simulink model "visual_line_follower_sac_residual"  (R2026a)
settings: Solver=FixedStepDiscrete  StopTime=40  FixedStep=MJ_StepTime  EnableMultiTasking=on
InitFcn:
  | run(fullfile(fileparts(get_param(bdroot,"FileName")),"runtime","init","configure_turtlebot3_visual_line_follower_paths.m"));
model workspace (MAT data in the model file):
  BaseLinearSpeed = 5
  BaseSpeedScale = 0.03
  Kd_Line = 0.35
  Ki_Line = 0
  Kp_Line = 5
  LocalPath_CurvatureGain = 0.04
  LocalPath_HeadingGain = 0.35
  LocalPath_LateralGain = 0.6
  LocalPath_LookaheadDistance = 0.2
  LocalPath_NumPoints = 30
  LocalPath_ROIFraction = 0.3
  MJ_StepTime = 0.002
  MJ_TargetLateralPosition = 0
  MaxAngularSpeed = 1.5
  MaxWheelSpeed = 7.9
  N_Line = 20
  OriginBot_ErrorScale = 500
  OriginBot_MaxSaturation = 0.3
  OriginBot_MinBrightness = 70
  OriginBot_MinPixels = 30
  OriginBot_ROIHeight = 45
  OriginBot_ROIStartFraction = 0.72
  SAC_Done_Steps = 100
  SAC_MaxDeltaOmega = 1
  SAC_MaxDeltaV = 1
  SAC_P_Lost = 10
  SAC_Q = 1
  SAC_Q_Heading = 0.5
  SAC_Q_Lateral = 0.5
  SAC_R = 0.1
  Safety_BrakeTime = 0.3
  Safety_CBFAlpha = 2
  Safety_CBFSingularTol = 0.001
  Safety_DirDeadband = 0.02
  Safety_EnableFilter = 1
  Safety_EnableSearch = 0
  Safety_HoldTime = 0.4
  Safety_LateralMax = 0.8
  Safety_MaxAccelOmega = 10
  Safety_MaxAccelV = 40
  Safety_MemLookahead = 0.25
  Safety_MemMaxAge = 8
  Safety_MemMinPoints = 3
  Safety_RecoverAlignCone = 0.785398163397
  Safety_RecoverGain = 1.5
  Safety_RecoverSpeedFrac = 0.25
  Safety_RecoverTimeout = 8
  Safety_ScanAmplitudes = [0.436332312999 0.872664625997 1.3962634016]
  Safety_ScanRate = 0.9
  Safety_ScanTimeout = 15
  Safety_ScanTolerance = 0.05
  Safety_SpeedBackoff = 0.3
  SteeringSign = -1
  TB3_WheelRadius = 0.033
  TB3_WheelSeparation = 0.16
  Ts_Control = 0.05
  Ts_Stop = 10
  Ts_Vision = 0.05
  TurtleBot3MuJoCoMap = "simple"
  TurtleBot3MuJoCoScene = ""
undefined symbols (not defined in the file or in its folder): lf_line_search, LF_Safety, lf_safety_filter, originbot_line_follower_debug_frame, originbot_sliding_window_path_generator
libraries: mjLib x1, slpidlib x1, rllib x1
settings Model: ExtModeTrigDuration=10000  Creator=HP  LastModifiedBy=kevin
settings SolverCC: PositivePriorityOrder=on
settings ConfigComp: CovMetricSettings=dswe

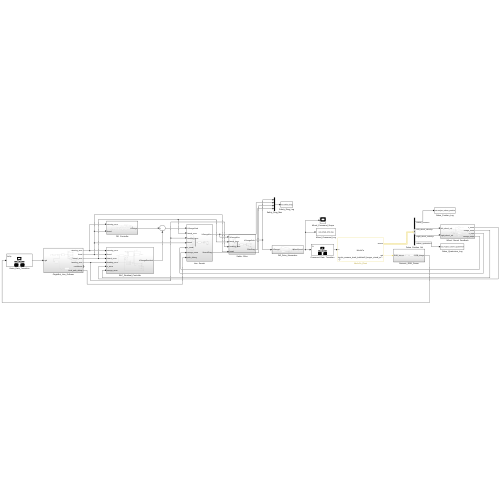
[thumbnail: Simulink's stored preview of the top-level diagram]
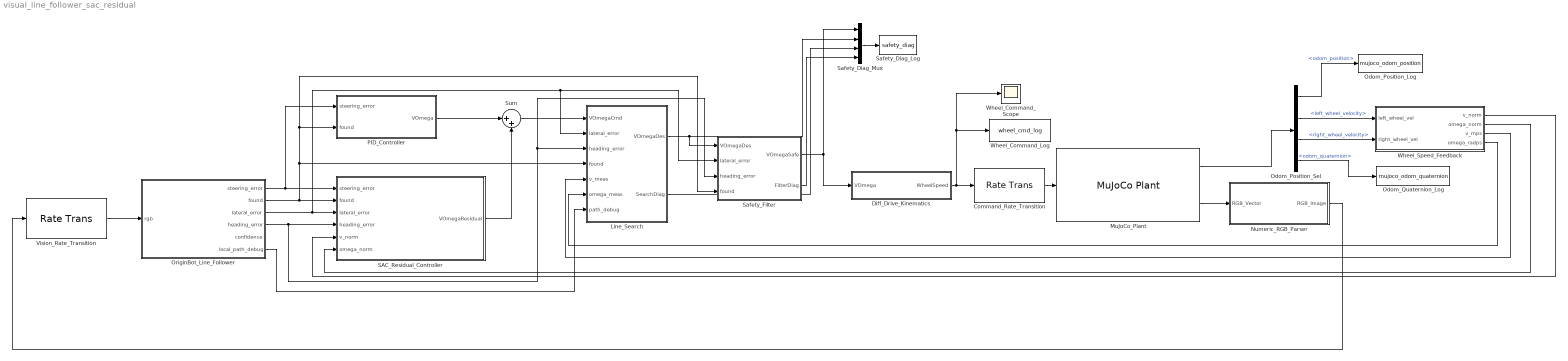
== system visual_line_follower_sac_residual ==
  Command_Rate_Transition : RateTransition  OutPortSampleTime=MJ_StepTime
  Diff_Drive_Kinematics : Subsystem  Description=Shared linear+angular velocity -> left/right wheel-speed converter. Input VOmega=[v;omega] is the summed PID+SAC velocity command (blk_124.y1); output WheelSpeed=[left;right] feeds SAC_PID_Sat (blk_125). Extracted 2026-07-21 from duplicated logic that used to live separately inside PID_Controller and SAC_Residual_Controller -- both now output [v;omega] instead of wheel speeds directly, and this is the ONE place the differential-drive kinematics conversion happens.
  Line_Search : Subsystem
  MuJoCo_Plant : mjLib/MuJoCo Plant  controlBus=[]  sensorBus=mj_bus_sensor_7979902499018342666  controlLength=[]  sensorLength=[]  rgbLength=[]  depthLength=[]  sampleTime=0.002  xmlFileRel=/media/kevin/ding/final_project/Sheffield/for_getting_started/src/simple_camera_pid/matlab/../model/mujoco/turtlebot3/simple_camera_track_turtlebot3_burger_visual_scene.xml  xmlFile=/media/kevin/ding/final_project/Sheffield/for_getting_started/src/simple_camera_pid/matlab/../model/mujoco/turtlebot3/simple_camera_track_turtlebot3_burger_visual_scene.xml  renderingType=Local  vsync=on  visualFPS=60  zoomLevel=1  znear=0.062275  zfar=311.3772  cameraSampleTime=Ts_Vision  rgbOutOption=on  depthOutOption=off  controlInterfaceType=Vector
      settings: SourceProductName=MuJoCo Simulator
  Numeric_RGB_Parser : Subsystem
  Odom_Position_Log : ToWorkspace  VariableName=mujoco_odom_position  SaveFormat=Timeseries  SampleTime=-1
  Odom_Position_Sel : BusSelector  OutputSignals=odom_position,left_wheel_velocity,right_wheel_velocity,odom_quaternion
  Odom_Quaternion_Log : ToWorkspace  VariableName=mujoco_odom_quaternion  SaveFormat=Timeseries  SampleTime=-1
  OriginBot_Line_Follower : Subsystem
  PID_Controller : Subsystem
  SAC_Residual_Controller : Subsystem
  Safety_Diag_Log : ToWorkspace  VariableName=safety_diag  SaveFormat=Structure With Time
  Safety_Diag_Mux : Mux
  Safety_Filter : Subsystem
  Sum : Sum  Inputs=|++
  Vision_Rate_Transition : RateTransition  OutPortSampleTime=Ts_Vision
  Wheel_Command_Log : ToWorkspace  VariableName=wheel_cmd_log  SaveFormat=Structure With Time
  Wheel_Command_Scope : Scope
  Wheel_Speed_Feedback : Subsystem
  wires:
  Diff_Drive_Kinematics/1(WheelSpeed) -> Wheel_Command_Scope/1, Wheel_Command_Log/1, Command_Rate_Transition/1
  Safety_Filter/1(VOmegaSafe) -> Safety_Diag_Mux/1, Diff_Drive_Kinematics/1(VOmega)
  Sum/1 -> Line_Search/1(VOmegaCmd)
  OriginBot_Line_Follower/3(lateral_error) -> SAC_Residual_Controller/3(lateral_error), Line_Search/2(lateral_error), Safety_Filter/2(lateral_error)
  OriginBot_Line_Follower/4(heading_error) -> SAC_Residual_Controller/4(heading_error), Safety_Filter/3(heading_error), Line_Search/3(heading_error)
  OriginBot_Line_Follower/2(found) -> Safety_Filter/4(found), PID_Controller/2(found), Line_Search/4(found), SAC_Residual_Controller/2(found)
  Wheel_Speed_Feedback/3(v_mps) -> Line_Search/5(v_meas)
  Wheel_Speed_Feedback/4(omega_radps) -> Line_Search/6(omega_meas)
  OriginBot_Line_Follower/6(local_path_debug) -> Line_Search/7(path_debug)
  Command_Rate_Transition/1 -> MuJoCo_Plant/1
  MuJoCo_Plant/2 -> Numeric_RGB_Parser/1(RGB_Vector)
  Odom_Position_Sel/1 -> Odom_Position_Log/1  "<odom_position>"
  MuJoCo_Plant/1 -> Odom_Position_Sel/1
  Odom_Position_Sel/4 -> Odom_Quaternion_Log/1  "<odom_quaternion>"
  Vision_Rate_Transition/1 -> OriginBot_Line_Follower/1(rgb)
  OriginBot_Line_Follower/1(steering_error) -> PID_Controller/1(steering_error), SAC_Residual_Controller/1(steering_error)
  Wheel_Speed_Feedback/1(v_norm) -> SAC_Residual_Controller/5(v_norm)
  Wheel_Speed_Feedback/2(omega_norm) -> SAC_Residual_Controller/6(omega_norm)
  Safety_Diag_Mux/1 -> Safety_Diag_Log/1
  Line_Search/1(VOmegaDes) -> Safety_Filter/1(VOmegaDes), Safety_Diag_Mux/2
  Line_Search/2(SearchDiag) -> Safety_Diag_Mux/3
  Safety_Filter/2(FilterDiag) -> Safety_Diag_Mux/4
  PID_Controller/1(VOmega) -> Sum/1
  SAC_Residual_Controller/1(VOmegaResidual) -> Sum/2
  Numeric_RGB_Parser/1(RGB_Image) -> Vision_Rate_Transition/1
  Odom_Position_Sel/2 -> Wheel_Speed_Feedback/1(left_wheel_vel)  "<left_wheel_velocity>"
  Odom_Position_Sel/3 -> Wheel_Speed_Feedback/2(right_wheel_vel)  "<right_wheel_velocity>"

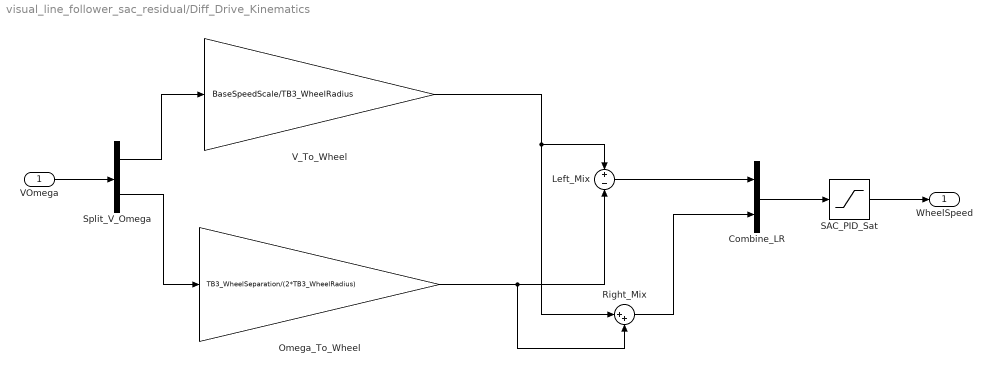
== system visual_line_follower_sac_residual/Diff_Drive_Kinematics ==
  VOmega : Inport
  Combine_LR : Mux  Inputs=2
  Left_Mix : Sum  Inputs=+-
  Omega_To_Wheel : Gain  Gain=TB3_WheelSeparation/(2*TB3_WheelRadius)
  Right_Mix : Sum  Inputs=|++
  SAC_PID_Sat : Saturate  UpperLimit=[MaxWheelSpeed; MaxWheelSpeed]  LowerLimit=-[MaxWheelSpeed; MaxWheelSpeed]
  Split_V_Omega : Demux  Outputs=2
  V_To_Wheel : Gain  Gain=BaseSpeedScale/TB3_WheelRadius
  WheelSpeed : Outport
  wires:
  VOmega/1 -> Split_V_Omega/1
  Split_V_Omega/1 -> V_To_Wheel/1
  Split_V_Omega/2 -> Omega_To_Wheel/1
  V_To_Wheel/1 -> Right_Mix/1, Left_Mix/1
  Combine_LR/1 -> SAC_PID_Sat/1
  Left_Mix/1 -> Combine_LR/1
  Omega_To_Wheel/1 -> Right_Mix/2, Left_Mix/2
  Right_Mix/1 -> Combine_LR/2
  SAC_PID_Sat/1 -> WheelSpeed/1

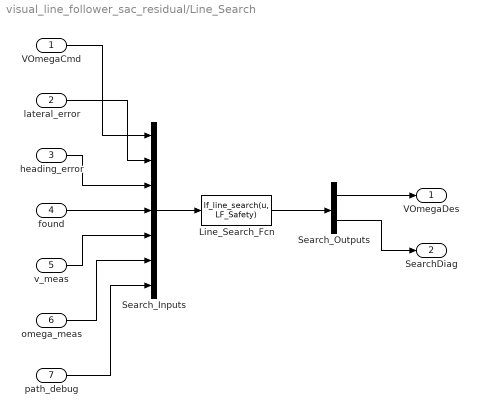
== system visual_line_follower_sac_residual/Line_Search ==
  VOmegaCmd : Inport
  lateral_error : Inport  Port=2
  heading_error : Inport  Port=3
  found : Inport  Port=4
  v_meas : Inport  Port=5
  omega_meas : Inport  Port=6
  path_debug : Inport  Port=7
  Line_Search_Fcn : MATLABFcn  MATLABFcn=lf_line_search(u, LF_Safety)  OutputDimensions=7  SampleTime=Ts_Control
  Search_Inputs : Mux  Inputs=7
  Search_Outputs : Demux  Outputs=[2 5]
  VOmegaDes : Outport
  SearchDiag : Outport  Port=2
  wires:
  Search_Outputs/2 -> SearchDiag/1
  Search_Outputs/1 -> VOmegaDes/1
  Line_Search_Fcn/1 -> Search_Outputs/1
  Search_Inputs/1 -> Line_Search_Fcn/1
  path_debug/1 -> Search_Inputs/7
  omega_meas/1 -> Search_Inputs/6
  v_meas/1 -> Search_Inputs/5
  found/1 -> Search_Inputs/4
  heading_error/1 -> Search_Inputs/3
  lateral_error/1 -> Search_Inputs/2
  VOmegaCmd/1 -> Search_Inputs/1

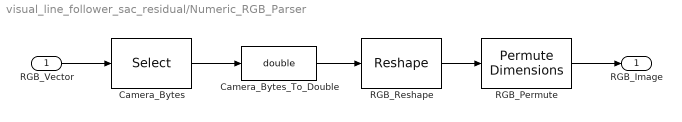
== system visual_line_follower_sac_residual/Numeric_RGB_Parser ==
  RGB_Vector : Inport
  Camera_Bytes : Selector  InputPortWidth=921601  IndexOptions=Index vector (dialog)  Indices=1:921600  OutputSizes=1
  Camera_Bytes_To_Double : DataTypeConversion  OutDataTypeStr=double
  RGB_Permute : PermuteDimensions  Order=[3 2 1]
  RGB_Reshape : Reshape  OutputDimensionality=Customize  OutputDimensions=[3,640,480]
  RGB_Image : Outport
  wires:
  Camera_Bytes_To_Double/1 -> RGB_Reshape/1
  RGB_Permute/1 -> RGB_Image/1
  RGB_Reshape/1 -> RGB_Permute/1
  Camera_Bytes/1 -> Camera_Bytes_To_Double/1
  RGB_Vector/1 -> Camera_Bytes/1

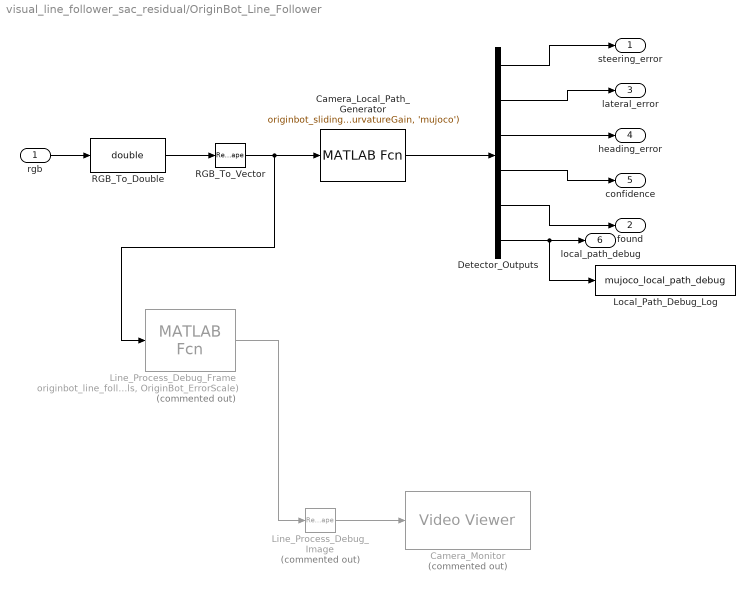
== system visual_line_follower_sac_residual/OriginBot_Line_Follower ==
  rgb : Inport
  Camera_Local_Path_Generator : MATLABFcn  MATLABFcn=originbot_sliding_window_path_generator(u, LocalPath_ROIFraction, LocalPath_NumPoints, OriginBot_MinBrightness, OriginBot_MaxSaturation, OriginBot_MinPixels, OriginBot_ErrorScale, LocalPath_LookaheadDistance, LocalPath_LateralGain, LocalPath_HeadingGain, LocalPath_CurvatureGain, 'mujoco')  OutputDimensions=72  OutputSignalType=real  SampleTime=Ts_Vision
  Camera_Monitor : VideoViewer  Commented=on  FigPos=[498 692 990 438]
  Detector_Outputs : Demux  Outputs=[1 1 1 1 1 67]
  Line_Process_Debug_Frame : MATLABFcn  Commented=on  MATLABFcn=originbot_line_follower_debug_frame(u, LocalPath_ROIFraction, LocalPath_NumPoints, OriginBot_MinBrightness, OriginBot_MaxSaturation, OriginBot_MinPixels, OriginBot_ErrorScale)
  Line_Process_Debug_Image : Reshape  Commented=on  OutputDimensionality=Customize  OutputDimensions=[480,640,3]
  Local_Path_Debug_Log : ToWorkspace  VariableName=mujoco_local_path_debug  SaveFormat=Timeseries  SampleTime=-1
  RGB_To_Double : DataTypeConversion  OutDataTypeStr=double
  RGB_To_Vector : Reshape  OutputDimensionality=Column vector (2-D)
  steering_error : Outport
  found : Outport  Port=2
  lateral_error : Outport  Port=3
  heading_error : Outport  Port=4
  confidence : Outport  Port=5
  local_path_debug : Outport  Port=6
  wires:
  Detector_Outputs/2 -> lateral_error/1
  rgb/1 -> RGB_To_Double/1
  RGB_To_Double/1 -> RGB_To_Vector/1
  Detector_Outputs/4 -> confidence/1
  Camera_Local_Path_Generator/1 -> Detector_Outputs/1
  Detector_Outputs/1 -> steering_error/1
  Detector_Outputs/3 -> heading_error/1
  Detector_Outputs/5 -> found/1
  Detector_Outputs/6 -> local_path_debug/1, Local_Path_Debug_Log/1
  RGB_To_Vector/1 -> Line_Process_Debug_Frame/1, Camera_Local_Path_Generator/1
  Line_Process_Debug_Frame/1 -> Line_Process_Debug_Image/1
  Line_Process_Debug_Image/1 -> Camera_Monitor/1

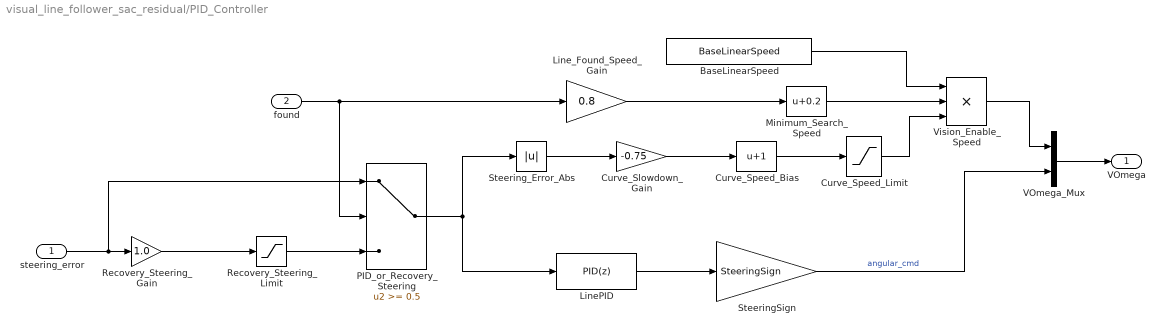
== system visual_line_follower_sac_residual/PID_Controller ==
  steering_error : Inport
  found : Inport  Port=2
  BaseLinearSpeed : Constant  Value=BaseLinearSpeed
  Curve_Slowdown_Gain : Gain  Gain=-0.75
  Curve_Speed_Bias : Bias  Bias=1
  Curve_Speed_Limit : Saturate  UpperLimit=1  LowerLimit=0.25
  LinePID : slpidlib/PID Controller  Controller=PID  Form=Parallel  TimeDomain=Discrete-time  UseExternalTs=off  SampleTime=Ts_Control  IntegratorMethod=Backward Euler  FilterMethod=Trapezoidal  ControllerParametersSource=internal  P=Kp_Line  I=Ki_Line  UseKiTs=off  D=Kd_Line  UseExternalDerivativeSource=off  N=N_Line  UseFilter=on  TunerSelectOption=Transfer Function Based (PID Tuner App)  InitialConditionSource=internal  InitialConditionForIntegrator=0  InitialConditionForFilter=0  DifferentiatorICPrevScaledInput=0  ExternalReset=none  TrackingMode=off  Kt=1  LimitOutput=on  SatLimitsSource=internal  UpperSaturationLimit=MaxAngularSpeed  LowerSaturationLimit=-MaxAngularSpeed  LinearizeAsGain=off  AntiWindupMode=back-calculation  Kb=1  LimitIntegrator=off  UpperIntegratorSaturationLimit=inf  LowerIntegratorSaturationLimit=-inf  POutMin=[]  POutMax=[]  IOutMin=[]  IOutMax=[]  DOutMin=[]  DOutMax=[]  NOutMin=[]  NOutMax=[]  SumOutMin=[]  SumOutMax=[]  SaturationOutMin=[]  SaturationOutMax=[]  PParamMin=[]  PParamMax=[]  IParamMin=[]  IParamMax=[]  DParamMin=[]  DParamMax=[]  NParamMin=[]  NParamMax=[]  KbParamMin=[]  KbParamMax=[]  KtParamMin=[]  KtParamMax=[]  KbOutMin=[]  KbOutMax=[]  KtOutMin=[]  KtOutMax=[]  IntegratorOutMin=[]  IntegratorOutMax=[]  FilterOutMin=[]  FilterOutMax=[]  SumI1OutMin=[]  SumI1OutMax=[]  SumI2OutMin=[]  SumI2OutMax=[]  SumI3OutMin=[]  SumI3OutMax=[]  SumI4OutMin=[]  SumI4OutMax=[]  SumDOutMin=[]  SumDOutMax=[]  DifferentiatorOutMin=[]  DifferentiatorOutMax=[]  FilterDiffOutCoefMin=[]  FilterDiffOutCoefMax=[]  ReciprocalOutMin=[]  ReciprocalOutMax=[]  SumDenOutMin=[]  SumDenOutMax=[]  SumNumOutMin=[]  SumNumOutMax=[]  DivideOutMin=[]  DivideOutMax=[]  UdiffTsProdOutMin=[]  UdiffTsProdOutMax=[]  NTsProdOutMin=[]  NTsProdOutMax=[]  UintegralTsProdOutMin=[]  UintegralTsProdOutMax=[]  UngainTsProdOutMin=[]  UngainTsProdOutMax=[]  ClampingZeroOutDataTypeStr=Inherit: Inherit via back propagation  ClampingZeroOutMin=[]  ClampingZeroOutMax=[]  FilterDenConstantOutDataTypeStr=Inherit: Inherit via back propagation  FilterDenConstantOutMin=[]  FilterDenConstantOutMax=[]  PCopyOutDataTypeStr=Inherit: Inherit via back propagation  PCopyOutMin=[]  PCopyOutMax=[]  NCopyOutDataTypeStr=Inherit: Inherit via back propagation  NCopyOutMin=[]  NCopyOutMax=[]  IntegratorContinuousStateAttributes=''  IntegratorStateMustResolveToSignalObject=off  IntegratorRTWStateStorageClass=Auto  FilterContinuousStateAttributes=''  FilterStateMustResolveToSignalObject=off  FilterRTWStateStorageClass=Auto  ParallelPVariant=InternalParameters  IdealPVariant=Disabled  IVariant=InternalParameters  DVariant=InternalParameters  IntegratorVariant=Discrete  SatVariant=Enabled  AWVariant=BackCalculation  PCopyVariant=Disabled  TRVariant=Disabled  FdbkBlocksVariant=Feedback  IdealPFdbkVariant=Passthrough  SatFdbkVariant=Enabled  DerivativeFilterVariant=TrapezoidalFilter  NVariant=InternalParameters  NCopyVariant=InternalParameters  FilterICVariant=InternalICsFilter  IntegratorICVariant=InternalICs  ExternalResetVariant=Disabled  TRSumVariant=Passthrough  SumFdbkVariant=Enabled  SumVariant=Sum_PID  TsampFilterVariant=InternalTs  TsampNgainVariant=Passthrough  TsampIntegralVariant=Disabled_SignalSpec  ExternalSaturationOutDataTypeStr=Inherit: Same as second input  DerivativeSourceVariant=ErrorSignal  PreIntVariant=InternalPreInt
      settings: LibrarySourceBlock=hdlsllib/Discrete/Discrete PID Controller
  Line_Found_Speed_Gain : Gain  Gain=0.8
  Minimum_Search_Speed : Bias  Bias=0.2
  PID_or_Recovery_Steering : Switch  Threshold=0.5
  Recovery_Steering_Gain : Gain  Gain=1.0
  Recovery_Steering_Limit : Saturate  UpperLimit=0.45  LowerLimit=-0.45
  SteeringSign : Gain  Gain=SteeringSign
  Steering_Error_Abs : Abs
  VOmega_Mux : Mux  Inputs=2
  Vision_Enable_Speed : Product  Inputs=***
  VOmega : Outport
  wires:
  VOmega_Mux/1 -> VOmega/1
  SteeringSign/1 -> VOmega_Mux/2  "angular_cmd"
  Vision_Enable_Speed/1 -> VOmega_Mux/1
  Curve_Speed_Limit/1 -> Vision_Enable_Speed/3
  BaseLinearSpeed/1 -> Vision_Enable_Speed/1
  LinePID/1 -> SteeringSign/1
  Curve_Speed_Bias/1 -> Curve_Speed_Limit/1
  Curve_Slowdown_Gain/1 -> Curve_Speed_Bias/1
  Steering_Error_Abs/1 -> Curve_Slowdown_Gain/1
  Line_Found_Speed_Gain/1 -> Minimum_Search_Speed/1
  Recovery_Steering_Limit/1 -> PID_or_Recovery_Steering/3
  Recovery_Steering_Gain/1 -> Recovery_Steering_Limit/1
  PID_or_Recovery_Steering/1 -> LinePID/1, Steering_Error_Abs/1
  found/1 -> PID_or_Recovery_Steering/2, Line_Found_Speed_Gain/1
  Minimum_Search_Speed/1 -> Vision_Enable_Speed/2
  steering_error/1 -> PID_or_Recovery_Steering/1, Recovery_Steering_Gain/1

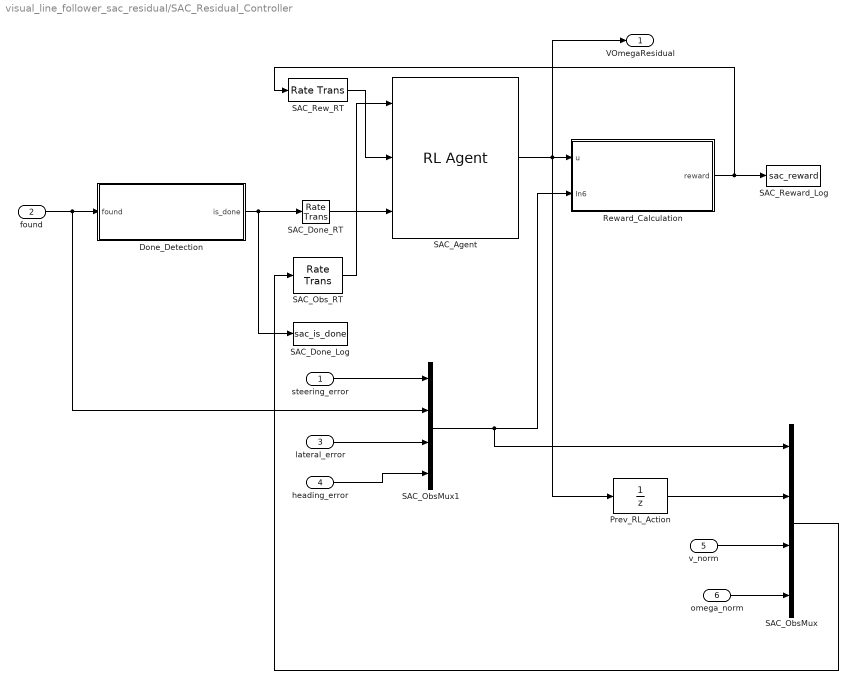
== system visual_line_follower_sac_residual/SAC_Residual_Controller ==
  steering_error : Inport
  found : Inport  Port=2
  lateral_error : Inport  Port=3
  heading_error : Inport  Port=4
  v_norm : Inport  Port=5
  omega_norm : Inport  Port=6
  Done_Detection : Subsystem
  Prev_RL_Action : UnitDelay  SampleTime=Ts_Control
  Reward_Calculation : Subsystem
  SAC_Agent : rllib/RL Agent  Agent=trainedAgent  ExternalActionAsInput=off  ProvideLastAction=off  ProvideCumRwd=off  TreatAsDirectFeedthrough=on  UseStrictObservationDataTypes=off
  SAC_Done_Log : ToWorkspace  VariableName=sac_is_done  SaveFormat=Timeseries  SampleTime=-1
  SAC_Done_RT : RateTransition  Integrity=off  Deterministic=off
  SAC_ObsMux : Mux
  SAC_ObsMux1 : Mux
  SAC_Obs_RT : RateTransition  Integrity=off  Deterministic=off
  SAC_Rew_RT : RateTransition  Integrity=off  Deterministic=off
  SAC_Reward_Log : ToWorkspace  VariableName=sac_reward  SaveFormat=Timeseries  SampleTime=-1
  VOmegaResidual : Outport
  wires:
  SAC_ObsMux/1 -> SAC_Obs_RT/1
  omega_norm/1 -> SAC_ObsMux/4
  found/1 -> SAC_ObsMux1/2, Done_Detection/1(found)
  Done_Detection/1(is_done) -> SAC_Done_Log/1, SAC_Done_RT/1
  Reward_Calculation/1(reward) -> SAC_Reward_Log/1, SAC_Rew_RT/1
  lateral_error/1 -> SAC_ObsMux1/3
  SAC_Done_RT/1 -> SAC_Agent/3
  SAC_Obs_RT/1 -> SAC_Agent/1
  SAC_Rew_RT/1 -> SAC_Agent/2
  steering_error/1 -> SAC_ObsMux1/1
  heading_error/1 -> SAC_ObsMux1/4
  SAC_ObsMux1/1 -> Reward_Calculation/2(In6), SAC_ObsMux/1
  SAC_Agent/1 -> VOmegaResidual/1, Reward_Calculation/1(u), Prev_RL_Action/1
  Prev_RL_Action/1 -> SAC_ObsMux/2
  v_norm/1 -> SAC_ObsMux/3

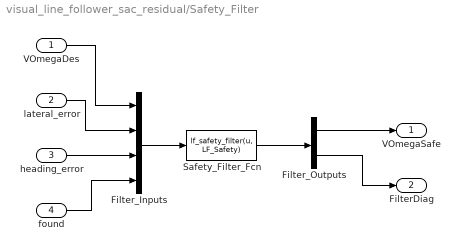
== system visual_line_follower_sac_residual/Safety_Filter ==
  VOmegaDes : Inport
  lateral_error : Inport  Port=2
  heading_error : Inport  Port=3
  found : Inport  Port=4
  Filter_Inputs : Mux
  Filter_Outputs : Demux  Outputs=[2 5]
  Safety_Filter_Fcn : MATLABFcn  MATLABFcn=lf_safety_filter(u, LF_Safety)  OutputDimensions=7  SampleTime=Ts_Control
  VOmegaSafe : Outport
  FilterDiag : Outport  Port=2
  wires:
  Filter_Outputs/2 -> FilterDiag/1
  Filter_Outputs/1 -> VOmegaSafe/1
  Safety_Filter_Fcn/1 -> Filter_Outputs/1
  Filter_Inputs/1 -> Safety_Filter_Fcn/1
  found/1 -> Filter_Inputs/4
  heading_error/1 -> Filter_Inputs/3
  lateral_error/1 -> Filter_Inputs/2
  VOmegaDes/1 -> Filter_Inputs/1

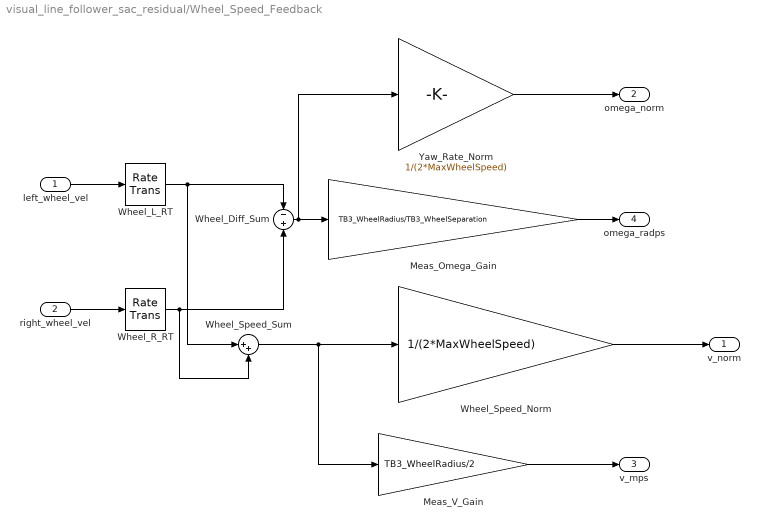
== system visual_line_follower_sac_residual/Wheel_Speed_Feedback ==
  left_wheel_vel : Inport
  right_wheel_vel : Inport  Port=2
  Meas_Omega_Gain : Gain  Gain=TB3_WheelRadius/TB3_WheelSeparation
  Meas_V_Gain : Gain  Gain=TB3_WheelRadius/2
  Wheel_Diff_Sum : Sum  Inputs=-+
  Wheel_L_RT : RateTransition  OutPortSampleTime=Ts_Control
  Wheel_R_RT : RateTransition  OutPortSampleTime=Ts_Control
  Wheel_Speed_Norm : Gain  Gain=1/(2*MaxWheelSpeed)
  Wheel_Speed_Sum : Sum  Inputs=|++
  Yaw_Rate_Norm : Gain  Gain=1/(2*MaxWheelSpeed)
  v_norm : Outport
  omega_norm : Outport  Port=2
  v_mps : Outport  Port=3
  omega_radps : Outport  Port=4
  wires:
  Meas_Omega_Gain/1 -> omega_radps/1
  Wheel_Speed_Sum/1 -> Wheel_Speed_Norm/1, Meas_V_Gain/1
  Yaw_Rate_Norm/1 -> omega_norm/1
  Wheel_R_RT/1 -> Wheel_Speed_Sum/2, Wheel_Diff_Sum/2
  Meas_V_Gain/1 -> v_mps/1
  Wheel_Speed_Norm/1 -> v_norm/1
  Wheel_Diff_Sum/1 -> Meas_Omega_Gain/1, Yaw_Rate_Norm/1
  Wheel_L_RT/1 -> Wheel_Speed_Sum/1, Wheel_Diff_Sum/1
  right_wheel_vel/1 -> Wheel_R_RT/1
  left_wheel_vel/1 -> Wheel_L_RT/1

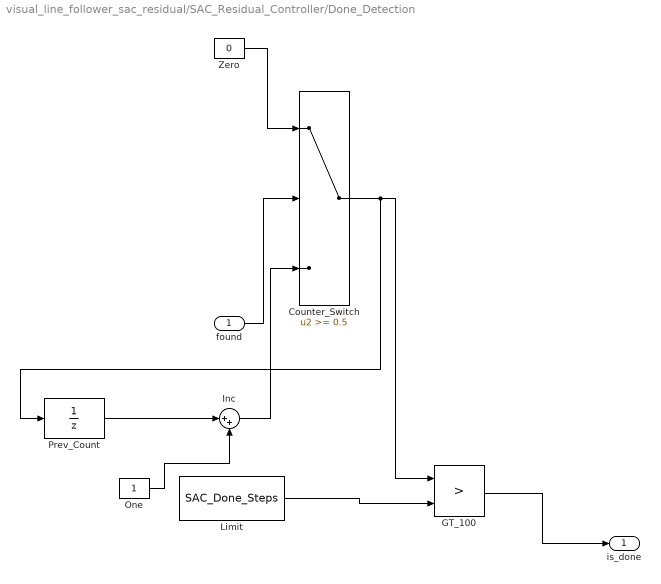
== system visual_line_follower_sac_residual/SAC_Residual_Controller/Done_Detection ==
  found : Inport
  Counter_Switch : Switch  Threshold=0.5  SaturateOnIntegerOverflow=off  InputSameDT=off
  GT_100 : RelationalOperator  Operator=>  OutDataTypeStr=boolean  RndMeth=Simplest  InputSameDT=off
  Inc : Sum  Inputs=|++
  Limit : Constant  Value=SAC_Done_Steps
  One : Constant
  Prev_Count : UnitDelay  SampleTime=Ts_Control
  Zero : Constant  Value=0
  is_done : Outport
  wires:
  Counter_Switch/1 -> GT_100/1, Prev_Count/1
  Limit/1 -> GT_100/2
  Inc/1 -> Counter_Switch/3
  Zero/1 -> Counter_Switch/1
  found/1 -> Counter_Switch/2
  One/1 -> Inc/2
  Prev_Count/1 -> Inc/1
  GT_100/1 -> is_done/1

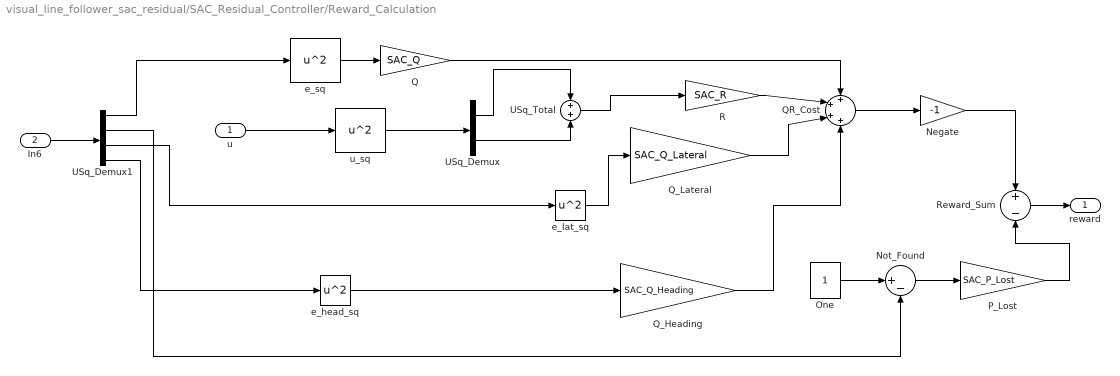
== system visual_line_follower_sac_residual/SAC_Residual_Controller/Reward_Calculation ==
  u : Inport
  In6 : Inport  Port=2
  Negate : Gain  Gain=-1
  Not_Found : Sum  Inputs=|+-
  One : Constant
  P_Lost : Gain  Gain=SAC_P_Lost
  Q : Gain  Gain=SAC_Q
  QR_Cost : Sum  Inputs=++++
  Q_Heading : Gain  Gain=SAC_Q_Heading
  Q_Lateral : Gain  Gain=SAC_Q_Lateral
  R : Gain  Gain=SAC_R
  Reward_Sum : Sum  Inputs=+-
  USq_Demux : Demux  Outputs=2
  USq_Demux1 : Demux
  USq_Total : Sum  Description=u is now the 2-D action [delta_omega; delta_v]; u_sq (blk_134) squares elementwise, this Demux+Sum reduces it to sum(u.^2) so R still penalizes total action energy across both dims.
  e_head_sq : Math  Operator=square
  e_lat_sq : Math  Operator=square
  e_sq : Math  Operator=square
  u_sq : Math  Operator=square
  reward : Outport
  wires:
  Q_Heading/1 -> QR_Cost/4
  Q_Lateral/1 -> QR_Cost/3
  e_head_sq/1 -> Q_Heading/1
  e_lat_sq/1 -> Q_Lateral/1
  USq_Total/1 -> R/1
  USq_Demux/2 -> USq_Total/2
  USq_Demux/1 -> USq_Total/1
  u_sq/1 -> USq_Demux/1
  Q/1 -> QR_Cost/1
  u/1 -> u_sq/1
  R/1 -> QR_Cost/2
  e_sq/1 -> Q/1
  One/1 -> Not_Found/1
  QR_Cost/1 -> Negate/1
  Not_Found/1 -> P_Lost/1
  P_Lost/1 -> Reward_Sum/2
  Negate/1 -> Reward_Sum/1
  Reward_Sum/1 -> reward/1
  In6/1 -> USq_Demux1/1
  USq_Demux1/1 -> e_sq/1
  USq_Demux1/2 -> Not_Found/2
  USq_Demux1/3 -> e_lat_sq/1
  USq_Demux1/4 -> e_head_sq/1
